simulink model "development_enviroment"  (R2021b)
settings: Solver=VariableStepAuto  StartTime=0.0  StopTime=100  RelTol=1e-3
undefined symbols (not defined in the file or in its folder): A, B, C, D, k1, k3, k_2, tau_1, tau_2, tau_3, zeta
settings Model: Creator=alefr  LastModifiedBy=alefr

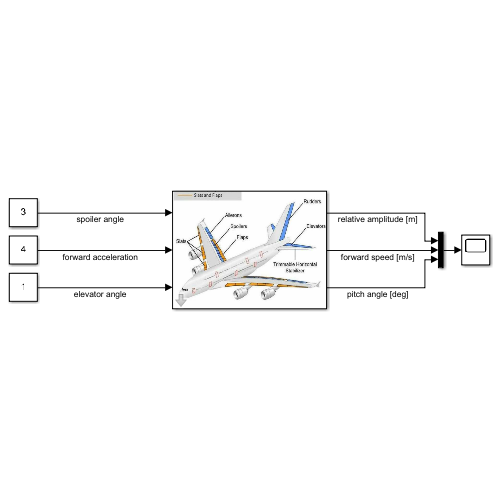
[thumbnail: Simulink's stored preview of the top-level diagram]
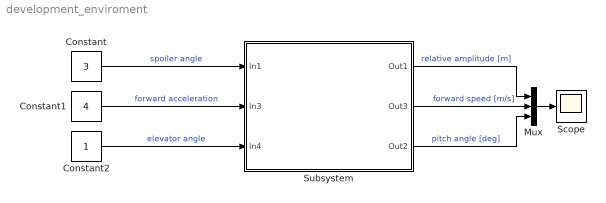
== system development_enviroment ==
  Constant : Constant  Value=3
  Constant1 : Constant  Value=4
  Constant2 : Constant
  Mux : Mux  Inputs=3
  Scope : Scope
  Subsystem : Subsystem  mask{k_2_param=mean(k_2), tau_1_param=mean(tau_1), tau_2_param=mean(tau_2), zeta_param=mean(zeta), tau_3_param=mean(tau_3)}
      mask prompts: k_2_param "k_2"; tau_1_param "tau_1"; tau_2_param "tau_2"; zeta_param "zeta"; tau_3_param "tau_3"
      mask Display: image('plane.png'); % Use "Edit Image" on toolstrip to change.
  wires:
  Constant/1 -> Subsystem/1(In1)  "spoiler angle"
  Constant1/1 -> Subsystem/2(In3)  "forward acceleration"
  Constant2/1 -> Subsystem/3(In4)  "elevator angle"
  Mux/1 -> Scope/1
  Subsystem/1(Out1) -> Mux/1  "relative amplitude [m]"
  Subsystem/3(Out2) -> Mux/3  "pitch angle [deg]"
  Subsystem/2(Out3) -> Mux/2  "forward speed [m/s]"

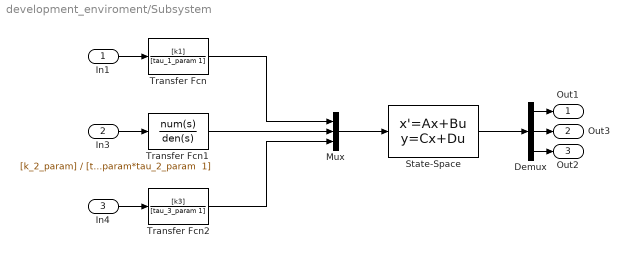
== system development_enviroment/Subsystem ==
  In1 : Inport
  In3 : Inport  Port=2
  In4 : Inport  Port=3
  Demux : Demux  Outputs=3
  Mux : Mux  Inputs=3
  State-Space : StateSpace  A=A  B=B  C=C  D=D  InitialCondition=0  ParameterTunability=Unconstrained
  Transfer Fcn : TransferFcn  Numerator=[k1]  Denominator=[tau_1_param 1]
  Transfer Fcn1 : TransferFcn  Numerator=[k_2_param]  Denominator="[tau_2_param^2  2*zeta_param*tau_2_param  1]"
  Transfer Fcn2 : TransferFcn  Numerator=[k3]  Denominator=[tau_3_param 1]
  Out1 : Outport
  Out3 : Outport  Port=2
  Out2 : Outport  Port=3
  wires:
  State-Space/1 -> Demux/1
  Transfer Fcn/1 -> Mux/1
  Transfer Fcn2/1 -> Mux/3
  Transfer Fcn1/1 -> Mux/2
  Demux/1 -> Out1/1
  Demux/2 -> Out3/1
  Mux/1 -> State-Space/1
  In4/1 -> Transfer Fcn2/1
  In3/1 -> Transfer Fcn1/1
  In1/1 -> Transfer Fcn/1
  Demux/3 -> Out2/1
